simulink model "AerodynamicMoment_wtf"  (R2023b)
settings: Solver=VariableStepAuto  StartTime=0.0  StopTime=Tfinal  RelTol=1e-3
model workspace: external: MATLAB File magConstants.m (data not in the file)
undefined symbols (not defined in the file or in its folder): areas, centroids, normalVectors, rcm
settings Model: Creator=kristopherriordan  LastModifiedBy=annahylbert

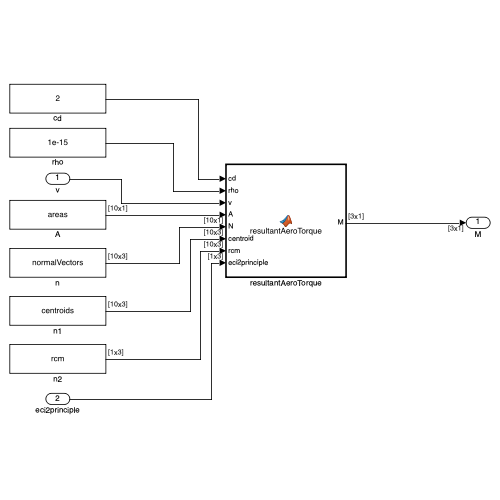
[thumbnail: Simulink's stored preview of the top-level diagram]
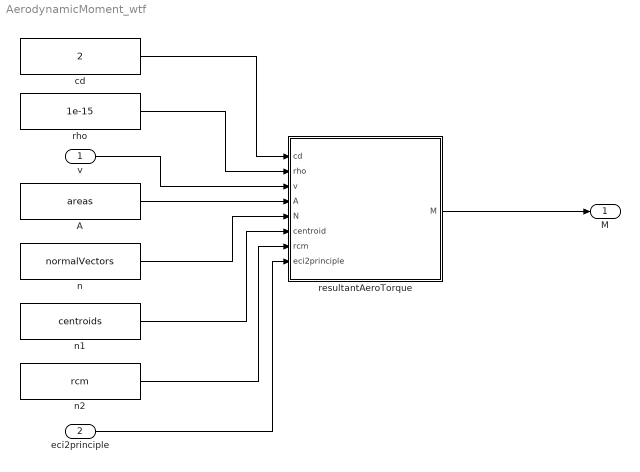
== system AerodynamicMoment_wtf ==
  v : Inport
  eci2principle : Inport  Port=2
  A : Constant  Value=areas  VectorParams1D=off
  cd : Constant  Value=2  VectorParams1D=off
  n : Constant  Value=normalVectors  VectorParams1D=off
  n1 : Constant  Value=centroids  VectorParams1D=off
  n2 : Constant  Value=rcm  VectorParams1D=off
  resultantAeroTorque : MATLAB Function  TreatAsAtomicUnit=on
  rho : Constant  Value=1e-15  VectorParams1D=off
  M : Outport
  wires:
  cd/1 -> resultantAeroTorque/1(cd)
  resultantAeroTorque/1(M) -> M/1
  v/1 -> resultantAeroTorque/3(v)
  n/1 -> resultantAeroTorque/5(N)
  rho/1 -> resultantAeroTorque/2(rho)
  A/1 -> resultantAeroTorque/4(A)
  eci2principle/1 -> resultantAeroTorque/8(eci2principle)
  n2/1 -> resultantAeroTorque/7(rcm)
  n1/1 -> resultantAeroTorque/6(centroid)

== matlab function AerodynamicMoment_wtf/resultantAeroTorque ==
  data: cd input; M output; rho input; v input; A input; N input; centroid input; rcm input; eci2principle input
function M = resultantAeroTorque(cd, rho, v, A, N, centroid, rcm, eci2principle)

n = size(A, 1);
v = eci2principle*v;
vUnit = v ./ norm(v);

M = zeros([3 1]);

N = A_ptob*N;


for i=1:n
    if dot(N(i, :), vUnit) > 0
        force = -0.5 .* cd .* rho .* norm(v)^2 .* A(i) .* dot(A_ptob*transpose(N(i, :)), vUnit) .* vUnit;
        M = M + cross(A_ptob*transpose(centroid(i, :) - rcm), force);
    end
end
